simulink model "modelo_LTI_3x3"  (R2023b)
settings: Solver=VariableStepAuto  StartTime=0.0  StopTime=10.0  RelTol=1e-3
values from neighbouring files (symbols this model uses):
  beq_nom = bm + bl_nom/r^2    (= 2.19444444444e-05)    [parametros_planta.m]    (also in params_subsistema_mecanico.m; sistema_completo_en_codigo.m)
  Cts = 0.818    [parametros_planta.m]    (also in params_subsistema_termico.m)
  Jeq_nom = Jm + Jl_nom/r^2    (= 1.97847222222e-05)    [params_subsistema_mecanico.m]    (also in sistema_completo_en_codigo.m)
  kg_eq_nom = g*kl_nom/r    (= 0.0204305208333)    [params_subsistema_mecanico.m]    (also in sistema_completo_en_codigo.m)
  L_q = 5.8e-3    (= 0.0058)    [controlador_foc_simulink.m]    (also in params_subsistema_electromagnetico.m; sistema_completo_en_codigo.m)
  lambda_m = 0.016    [controlador_foc_simulink.m]    (also in parametros_planta.m; params_subsistema_electromagnetico.m; sistema_completo_en_codigo.m)
  Pp = 3    [controlador_foc_simulink.m]    (also in parametros_planta.m; params_subsistema_electromagnetico.m; sistema_completo_en_codigo.m)
  r = 120.0    (= 120)    [controlador_foc_simulink.m]    (also in parametros_planta.m; params_subsistema_mecanico.m; sistema_completo_en_codigo.m)
  Rs_REF = 1.02    [controlador_foc_simulink.m]    (also in parametros_planta.m; params_subsistema_termico.m; sistema_completo_en_codigo.m)
  Rts_amb = 146.7    [parametros_planta.m]    (also in params_subsistema_termico.m)
  Tamb = Tamb_max    (= 40)    [parametros_planta.m]    (also in params_subsistema_termico.m; sistema_completo_en_codigo.m)
settings Model: Creator=Gabriel  LastModifiedBy=Gabriel

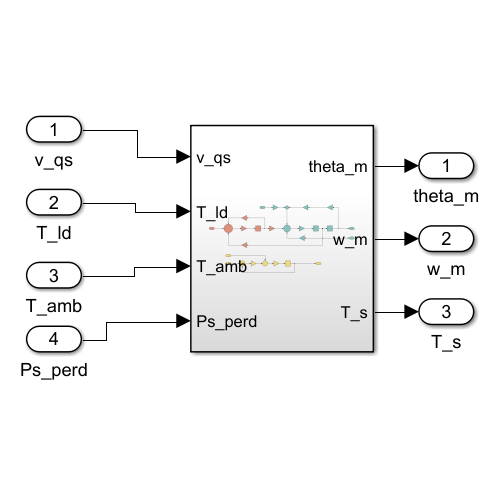
[thumbnail: Simulink's stored preview of the top-level diagram]
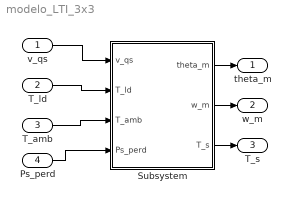
== system modelo_LTI_3x3 ==
  v_qs : Inport
  T_ld : Inport  Port=2
  T_amb : Inport  Port=3
  Ps_perd : Inport  Port=4
  Subsystem : Subsystem
  theta_m : Outport
  w_m : Outport  Port=2
  T_s : Outport  Port=3
  wires:
  v_qs/1 -> Subsystem/1(v_qs)
  T_ld/1 -> Subsystem/2(T_ld)
  T_amb/1 -> Subsystem/3(T_amb)
  Ps_perd/1 -> Subsystem/4(Ps_perd)
  Subsystem/1(theta_m) -> theta_m/1
  Subsystem/2(w_m) -> w_m/1
  Subsystem/3(T_s) -> T_s/1

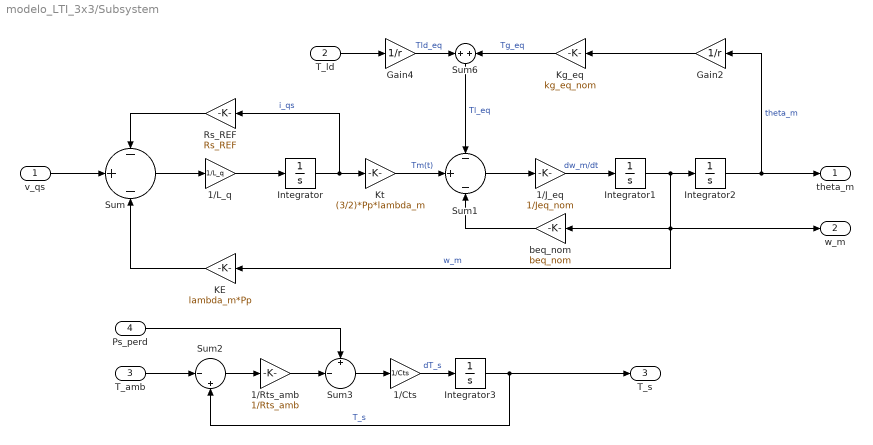
== system modelo_LTI_3x3/Subsystem ==
  v_qs : Inport
  T_ld : Inport  Port=2
  T_amb : Inport  Port=3
  Ps_perd : Inport  Port=4
  1/Cts : Gain  Gain=1/Cts
  1/J_eq : Gain  Gain=1/Jeq_nom
  1/L_q : Gain  Gain=1/L_q
  1/Rts_amb : Gain  Gain=1/Rts_amb
  Gain2 : Gain  Gain=1/r
  Gain4 : Gain  Gain=1/r
  Integrator : Integrator
  Integrator1 : Integrator
  Integrator2 : Integrator
  Integrator3 : Integrator  InitialCondition=Tamb
  KE : Gain  Gain=lambda_m*Pp
  Kg_eq : Gain  Gain=kg_eq_nom
  Kt : Gain  Gain=(3/2)*Pp*lambda_m
  Rs_REF : Gain  Gain=Rs_REF
  Sum : Sum  Inputs=-||+||-
  Sum1 : Sum  Inputs=-||+||-
  Sum2 : Sum  Inputs=||-|+
  Sum3 : Sum  Inputs=+|-||
  Sum6 : Sum  Inputs=+|+
  beq_nom : Gain  Gain=beq_nom
  theta_m : Outport
  w_m : Outport  Port=2
  T_s : Outport  Port=3
  wires:
  beq_nom/1 -> Sum1/3
  Kt/1 -> Sum1/2  "Tm(t)"
  1/J_eq/1 -> Integrator1/1  "dw_m/dt"
  Sum3/1 -> 1/Cts/1
  Sum6/1 -> Sum1/1  "Tl_eq"
  Gain4/1 -> Sum6/1  "Tld_eq"
  Integrator1/1 -> w_m/1, KE/1, beq_nom/1, Integrator2/1  "w_m"
  v_qs/1 -> Sum/2
  Sum/1 -> 1/L_q/1
  Integrator/1 -> Kt/1, Rs_REF/1  "i_qs"
  1/Rts_amb/1 -> Sum3/2
  Integrator3/1 -> T_s/1, Sum2/2  "T_s"
  Gain2/1 -> Kg_eq/1
  1/Cts/1 -> Integrator3/1  "dT_s"
  Integrator2/1 -> theta_m/1, Gain2/1  "theta_m"
  1/L_q/1 -> Integrator/1
  Ps_perd/1 -> Sum3/1
  Rs_REF/1 -> Sum/1
  Sum2/1 -> 1/Rts_amb/1
  Sum1/1 -> 1/J_eq/1
  KE/1 -> Sum/3
  T_ld/1 -> Gain4/1
  T_amb/1 -> Sum2/1
  Kg_eq/1 -> Sum6/2  "Tg_eq"
